simulink model "CentroInfladoLlantas"  (R2026a)
settings: Solver=VariableStepAuto  StopTime=480
undefined symbols (not defined in the file): m, n
settings Model: Creator=aboudonji  LastModifiedBy=aboudonji

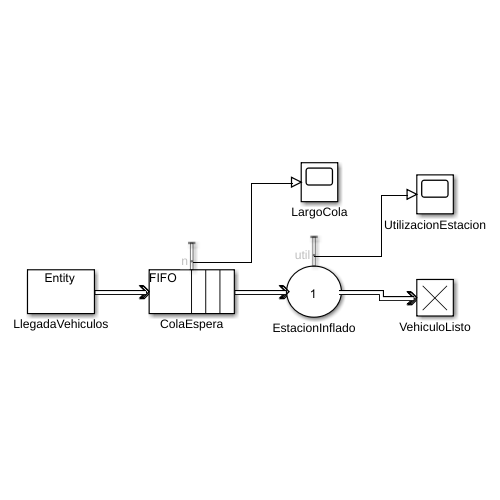
[thumbnail: Simulink's stored preview of the top-level diagram]
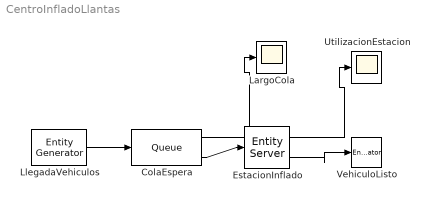
== system CentroInfladoLlantas ==
  ColaEspera : Queue  InputPortMessageModes=m  OutputPortMessageModes=n,m  NumberEntitiesInBlock=on
      settings: OutputPortMap=o1,o5
  EstacionInflado : EntityServer  InputPortMessageModes=m  OutputPortMessageModes=n,m  Capacity=1  ServiceTimeSource=MATLAB action  ServiceTimeAction=dt = -3*log(rand(1,1));  Utilization=on
      settings: OutputPortMap=o5,o9
  LargoCola : Scope
  LlegadaVehiculos : EntityGenerator  OutputPortMessageModes=m  TimeSource=MATLAB action  IntergenerationTimeAction=dt = -5*log(rand(1,1));  EntityType=Structured  EntityTypeName=Entity
  UtilizacionEstacion : Scope
  VehiculoListo : EntityTerminator  InputPortMessageModes=m
  wires:
  LlegadaVehiculos/1 -> ColaEspera/1
  ColaEspera/2 -> EstacionInflado/1
  EstacionInflado/2 -> VehiculoListo/1
  ColaEspera/1 -> LargoCola/1
  EstacionInflado/1 -> UtilizacionEstacion/1
